simulink model "convertidor_inversor"  (R2022b)
settings: Solver=VariableStepAuto  StartTime=0.0  StopTime=1  RelTol=1e-3
InitFcn:
  | Ts = 100e-6;
StartFcn:
  | Ts = 100e-6;
undefined symbols (not defined in the file): Ion, Lithium
libraries: spsIGBTDiodeLib x8, slpidlib x7, spsCurrentMeasurementLib x5, spsVoltageMeasurementLib x5, spsThreePhaseSeriesRLCBranchLib x5, spsSeriesRLCBranchLib x4, spsAlphaBetaZerotodq0Lib x3, simulink x3, spsabctoAlphaBetaZeroLib x3, spsDCVoltageSourceLib x2, spsThreePhaseVIMeasurementLib x2, spsBatteryLib x1
(part 1 of 2)
settings Model: Creator=JGC  LastModifiedBy=ATV
settings SolverCC: AlgebraicLoopSolver=TrustRegion
settings DataIOCC: ReturnWorkspaceOutputs=off
settings DebuggingCC: UnconnectedInputMsg=warning  UnconnectedOutputMsg=warning  UnconnectedLineMsg=warning  SFMachineParentedDataDiag=warning
settings ModelReferenceCC: EnableRefExpFcnMdlSchedulingChecks=on
settings RTWCC: DLArmComputeVersion=19.05

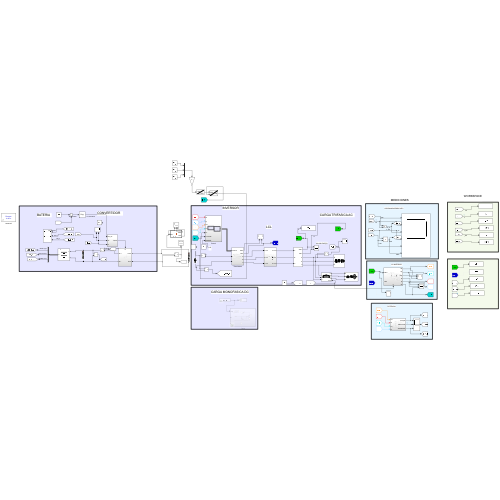
[thumbnail: Simulink's stored preview of the top-level diagram]
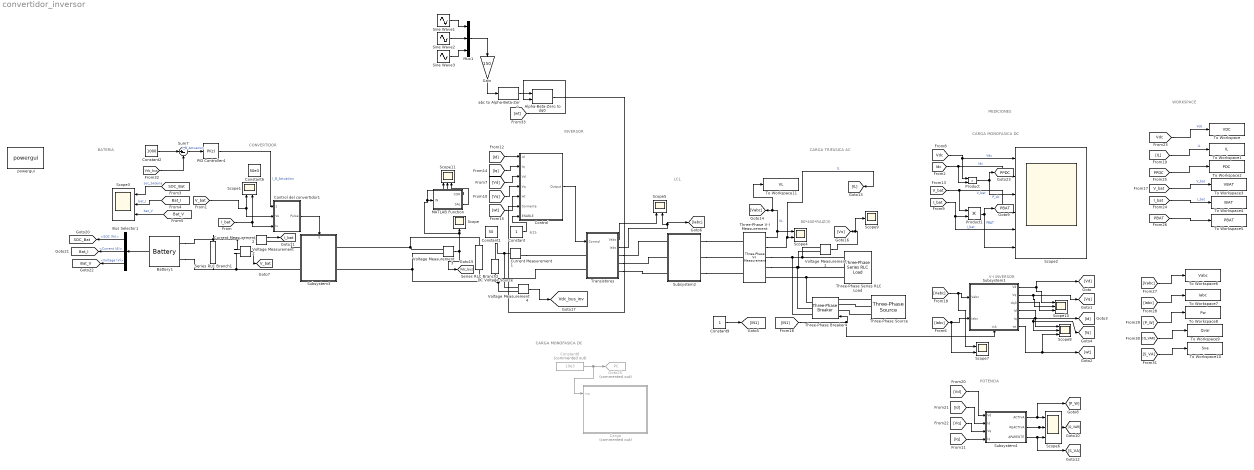
== system convertidor_inversor ==
  note: CARGA MONOFASICA DC
  note: CARGA TRIFASICA AC
  note: LCL
  note: INVERSOR
  note: MEDICIONES
  note: CARGA MONOFASICA DC
  note: BATERIA
  note: 80*400*RAIZ(3)
  note: 615
  note: POTENCIA
  note: V-I INVERSOR
  note: CONVERTIDOR
  note: WORKSPACE
  Alpha-Beta-Zero to dq0 : spsAlphaBetaZerotodq0Lib/Alpha-Beta-Zero to dq0  Alignment=90 degrees behind phase A axis
  Battery1 : spsBatteryLib/Battery  BatType=Lithium-Ion  ShowTempParam=off  ThermalPreset=no  ShowAgeParam=off  NomV=Battery.Nominal_voltage  NomQ=Battery.Rated_capacity  SOC=Battery.inicial_state_of_charge  Batt_Tr=Battery.response_time  PresetModel=on  MaxQ=200  MinV=384  FullV=595.9614  Dis_rate=86.9565  R=0.0256  Normal_OP=180.8696  expZone="[553.1576      9.826087]"  current=[6.5 7 100]  Units=Time  Tci=20  NomT=20  T2=-30  MaxQ2=4.8  FullV2=7.1  Normal_OP2=5.655  expZone2="[6.58           1]"  Rca=0.6  ti=2000  Dp=0  Neq0=0  Tsim=1e6  Ta1=25  Qeol=5.4*0.9  Reol=0.013333*1.2  Char_age=[2.3478, 3]  Dis_age=[2.3478, 10]  N1=1500  N2=10500  N3=1000  N4=1400  Ta2=45  N5=950
      settings: LibrarySourceBlock=electricdrivelib/Extra Sources/Battery
  Bus Selector1 : BusSelector  OutputSignals=SOC (%),Current (A),Voltage (V)
  Carga : Subsystem  Commented=on
  Constant : Constant
  Constant1 : Constant  Value=50
  Constant2 : Constant  Value=1000
  Constant6 : Constant  Value=50e3
  Constant8 : Constant  Commented=on  Value=10e3
  Constant9 : Constant
  "Control " : Subsystem
  Control del convertidor1 : Subsystem
  Current Measurement1 : spsCurrentMeasurementLib/Current Measurement  PhasorSimulation=off  OutputType=Complex  PSBequivalent=0
  Current Measurement2 : spsCurrentMeasurementLib/Current Measurement  PhasorSimulation=off  OutputType=Complex  PSBequivalent=0
  DC Voltage Source : spsDCVoltageSourceLib/DC Voltage Source  Amplitude=615  Measurements=None
  Gain : Gain  Gain=150
  Goto25 : Goto  Commented=on  GotoTag=PC  TagVisibility=global
  MATLAB Function : MATLAB Function  TreatAsAtomicUnit=on
  Mux1 : Mux  Inputs=3
  PID Controller4 : slpidlib/PID Controller  Controller=PI  Form=Parallel  TimeDomain=Discrete-time  UseExternalTs=off  SampleTime=Ts  IntegratorMethod=Forward Euler  FilterMethod=Forward Euler  ControllerParametersSource=internal  P=60  I=600  UseKiTs=off  D=0  N=100  UseFilter=on  TunerSelectOption=Transfer Function Based (PID Tuner App)  InitialConditionSource=internal  InitialConditionForIntegrator=0  InitialConditionForFilter=0  DifferentiatorICPrevScaledInput=0  ExternalReset=none  TrackingMode=off  Kt=1  LimitOutput=off  SatLimitsSource=internal  UpperSaturationLimit=0.95  LowerSaturationLimit=0  LinearizeAsGain=on  AntiWindupMode=clamping  Kb=1  LimitIntegrator=off  UpperIntegratorSaturationLimit=inf  LowerIntegratorSaturationLimit=-inf  POutMin=[]  POutMax=[]  IOutMin=[]  IOutMax=[]  DOutMin=[]  DOutMax=[]  NOutMin=[]  NOutMax=[]  SumOutMin=[]  SumOutMax=[]  SaturationOutMin=[]  SaturationOutMax=[]  PParamMin=[]  PParamMax=[]  IParamMin=[]  IParamMax=[]  DParamMin=[]  DParamMax=[]  NParamMin=[]  NParamMax=[]  KbParamMin=[]  KbParamMax=[]  KtParamMin=[]  KtParamMax=[]  KbOutMin=[]  KbOutMax=[]  KtOutMin=[]  KtOutMax=[]  IntegratorOutMin=[]  IntegratorOutMax=[]  FilterOutMin=[]  FilterOutMax=[]  SumI1OutMin=[]  SumI1OutMax=[]  SumI2OutMin=[]  SumI2OutMax=[]  SumI3OutMin=[]  SumI3OutMax=[]  SumI4OutMin=[]  SumI4OutMax=[]  SumDOutMin=[]  SumDOutMax=[]  DifferentiatorOutMin=[]  DifferentiatorOutMax=[]  FilterDiffOutCoefMin=[]  FilterDiffOutCoefMax=[]  ReciprocalOutMin=[]  ReciprocalOutMax=[]  SumDenOutMin=[]  SumDenOutMax=[]  SumNumOutMin=[]  SumNumOutMax=[]  DivideOutMin=[]  DivideOutMax=[]  UdiffTsProdOutMin=[]  UdiffTsProdOutMax=[]  NTsProdOutMin=[]  NTsProdOutMax=[]  UintegralTsProdOutMin=[]  UintegralTsProdOutMax=[]  UngainTsProdOutMin=[]  UngainTsProdOutMax=[]  ClampingZeroOutDataTypeStr=Inherit: Inherit via back propagation  ClampingZeroOutMin=[]  ClampingZeroOutMax=[]  FilterDenConstantOutDataTypeStr=Inherit: Inherit via back propagation  FilterDenConstantOutMin=[]  FilterDenConstantOutMax=[]  PCopyOutDataTypeStr=Inherit: Inherit via back propagation  PCopyOutMin=[]  PCopyOutMax=[]  NCopyOutDataTypeStr=Inherit: Inherit via back propagation  NCopyOutMin=[]  NCopyOutMax=[]  IntegratorContinuousStateAttributes=''  IntegratorStateMustResolveToSignalObject=off  IntegratorRTWStateStorageClass=Auto  FilterContinuousStateAttributes=''  FilterStateMustResolveToSignalObject=off  FilterRTWStateStorageClass=Auto  ParallelPVariant=InternalParameters  IdealPVariant=Disabled  IVariant=InternalParameters  DVariant=Disabled  IntegratorVariant=Discrete  SatVariant=Disabled  AWVariant=Passthrough  PCopyVariant=Disabled  TRVariant=Disabled  FdbkBlocksVariant=Forward  IdealPFdbkVariant=Disabled  SatFdbkVariant=Disabled  DerivativeFilterVariant=Disabled  NVariant=Disabled  NCopyVariant=Disabled_SignalSpec  FilterICVariant=Disabled  IntegratorICVariant=InternalICs  ExternalResetVariant=Disabled  TRSumVariant=Passthrough  SumFdbkVariant=Disabled  SumVariant=Sum_PI  TsampFilterVariant=InternalTs  TsampNgainVariant=Passthrough  TsampIntegralVariant=Passthrough  ExternalSaturationOutDataTypeStr=Inherit: Same as second input
  Product : Product
  Product1 : Product
  Scope : Scope
  Scope{1,4..5,7} (4 alike) : Scope  NumInputPorts=2
  Scope{3,6,8,10..11} (5 alike) : Scope  NumInputPorts=3
  Scope2 : Scope  NumInputPorts=6
  Scope9 : Scope
  Series RLC Branch1 : spsSeriesRLCBranchLib/Series RLC Branch  LConnTagsString=__new0  RConnTagsString=__new0  BranchType=RC  Resistance=0.3  Inductance=1e-3  SetiL0=off  InitialCurrent=0  Capacitance=1e-6  Setx0=on  InitialVoltage=512  Measurements=None
  Series RLC Branch2 : spsSeriesRLCBranchLib/Series RLC Branch  LConnTagsString=__new0  RConnTagsString=__new0  BranchType=C  Resistance=0.2  Inductance=1e-3  SetiL0=off  InitialCurrent=0  Capacitance=1000e-6  Setx0=on  InitialVoltage=400  Measurements=None
  Sine Wave1 : Sin  Frequency=2*pi*50  SampleTime=Ts
  Sine Wave2 : Sin  Frequency=2*pi*50  Phase=-120*2*pi/360  SampleTime=Ts
  Sine Wave3 : Sin  Frequency=2*pi*50  Phase=120*2*pi/360  SampleTime=Ts
  Subsystem1 : Subsystem
      settings: PortSchema="{\"entries\":[{\"content\":{\"sides\":[{\"content\":{\"connectorIds\":[\"In1\",\"In2\"]},\"type\":\"ConnectorPlacement.EquallySpacedRectSide\",\"uuid\":\"6be78711-4f19-4216-8280-237e362f2f67\"},{\"content\":{\"connectorIds\":[\"Out1\",\"Out2\",\"Out3\",\"Out4\",\"Out5\",\"Out6\"],\"side\":\"RIGHT\"},\"type\":\"ConnectorPlacement.EquallySpacedRectSide\",\"uuid\":\"8d48e04c-a554-48a1-8f05-ac010a5803c1\"},{\"content\":{\"connectorIds\":[],\"side\":\"TOP\"},\"type\":\"ConnectorPlacement.EquallySpacedRectSide\",\"uuid\":\"0ffbfd7d-1930-4ad5-9982-8469f3a97706\"},{\"content\":{\"connectorIds\":[\"In3\"],\"side\":\"BOTTOM\"},\"type\":\"ConnectorPlacement.EquallySpacedRectSide\",\"uuid\":\"6c965d76-c4d6-4dc7-a84d-e506f80fe6fe\"}]},\"type\":\"ConnectorPlacement.EquallySpacedConnector\",\"uuid\":\"0d915b79-5115-4aee-9d8b-435daa5fa966\"}],\"packageUris\":[\"http://schema.mathworks.com/mf0/Connector/R2020b\"],\"version\":\"1.0\"}"
  Subsystem2 : Subsystem
  Subsystem3 : Subsystem
      settings: PortSchema="{\"entries\":[{\"content\":{\"sides\":[{\"content\":{\"connectorIds\":[\"LConn1\",\"LConn2\"]},\"type\":\"ConnectorPlacement.EquallySpacedRectSide\",\"uuid\":\"7a980847-0fd3-4a52-ae22-59cd2a1ed559\"},{\"content\":{\"connectorIds\":[\"RConn1\",\"RConn2\"],\"side\":\"RIGHT\"},\"type\":\"ConnectorPlacement.EquallySpacedRectSide\",\"uuid\":\"85effeeb-73a6-4b0a-b51b-5eb0082317ff\"},{\"content\":{\"connectorIds\":[\"In1\"],\"side\":\"TOP\"},\"type\":\"ConnectorPlacement.EquallySpacedRectSide\",\"uuid\":\"eb55fae0-79ad-414f-ab96-49c332138803\"},{\"content\":{\"connectorIds\":[],\"side\":\"BOTTOM\"},\"type\":\"ConnectorPlacement.EquallySpacedRectSide\",\"uuid\":\"1fd972ff-419a-4657-8ea4-57d89be2b868\"}]},\"type\":\"ConnectorPlacement.EquallySpacedConnector\",\"uuid\":\"1807473d-fd42-44e0-a7e4-668a7bf21429\"}],\"packageUris\":[\"http://schema.mathworks.com/mf0/Connector/R2020b\"],\"version\":\"1.0\"}"
  Subsystem4 : Subsystem
  Sum7 : Sum  Inputs=|+-
  Three-Phase Series RLC Load : spsThreePhaseSeriesRLCLoadLib/Three-Phase Series RLC Load  LConnTagsString=A|B|C  Configuration=Y (grounded)  NominalVoltage=400  Vabc=[1e3 1e3 1e3]  Vabcp=[1e3 1e3 1e3]  NominalFrequency=50  UnbalancedPower=off  ActivePower=50e3  InductivePower=100  CapacitivePower=100  Pabc=[10e3 9e3 11e3]  QLabc=[100 90 110]  QCabc=[100 90 110]  Pabcp=[10e3 9e3 11e3]  QLabcp=[100 90 110]  QCabcp=[100 90 110]  Measurements=None  LoadType=constant Z
  Three-Phase V-I Measurement : spsThreePhaseVIMeasurementLib/Three-Phase V-I Measurement  VoltageMeasurement=phase-to-phase  SetLabelV=off  LabelV=Vabc  Vpu=off  VpuLL=off  CurrentMeasurement=yes  SetLabelI=off  LabelI=Iabc  Ipu=off  Pbase=100e6  Vbase=500e3  OutputType=Complex  PhasorSimulation=off  PSBequivalent=0
  Three-Phase Breaker4 : spsThreePhaseBreakerLib/Three-Phase Breaker  InitialState=closed  SwitchA=on  SwitchB=on  SwitchC=on  SwitchTimes="[1/60  5/60]"  External=on  BreakerResistance=0.01  SnubberResistance=1e6  SnubberCapacitance=inf  Measurements=None
  Three-Phase Source : spsThreePhaseSourceLib/Three-Phase Source  InternalConnection=Y  VoltagePhases=off  Voltage=400  PhaseAngle=0  Voltage_phases=[25e3 25e3 25e3]/sqrt(3)  PhaseAngles_phases=[0 -120 +120]  Frequency=50  NonIdealSource=on  SpecifyImpedance=off  Resistance=0.0001e-3  Inductance=0.0001e-9  ShortCircuitLevel=100e6  BaseVoltage=400  XRratio=7  BusType=swing  Pref=10e3  Qref=0  Prefabc=[10e3, 10e3, 10e3]  Qrefabc=[0, 0, 0]  Qmin=-inf  Qmax=inf
  To Workspace : ToWorkspace  VariableName=VDC  SaveFormat=Timeseries  SampleTime=-1
  To Workspace1 : ToWorkspace  VariableName=IL  SaveFormat=Timeseries  SampleTime=-1
  To Workspace10 : ToWorkspace  VariableName=Sva  SaveFormat=Timeseries  SampleTime=-1
  To Workspace11 : ToWorkspace  VariableName=VL  SaveFormat=Timeseries  SampleTime=-1
  To Workspace2 : ToWorkspace  VariableName=PDC  SaveFormat=Timeseries  SampleTime=-1
  To Workspace3 : ToWorkspace  VariableName=VBAT  SaveFormat=Timeseries  SampleTime=-1
  To Workspace4 : ToWorkspace  VariableName=IBAT  SaveFormat=Timeseries  SampleTime=-1
  To Workspace5 : ToWorkspace  VariableName=PBAT  SaveFormat=Timeseries  SampleTime=-1
  To Workspace6 : ToWorkspace  VariableName=Vabc  SaveFormat=Timeseries  SampleTime=-1
  To Workspace7 : ToWorkspace  VariableName=Iabc  SaveFormat=Timeseries  SampleTime=-1
  To Workspace8 : ToWorkspace  VariableName=Pw  SaveFormat=Timeseries  SampleTime=-1
  To Workspace9 : ToWorkspace  VariableName=Qvar  SaveFormat=Timeseries  SampleTime=-1
  Transistores : Subsystem
  Voltage Measurement{1..4} (4 alike) : spsVoltageMeasurementLib/Voltage Measurement  PhasorSimulation=off  OutputType=Complex  PSBequivalent=0
  abc to Alpha-Beta-Zero : spsabctoAlphaBetaZeroLib/abc to Alpha-Beta-Zero
  powergui : sps_lib/powergui  Priority=1  SimulationMode=Discrete  SampleTime=1e-5  frequency=60  Iterations=50  frequencyindice=0  Pbase=100e6  ErrMax=1e-4  UnitsV=kV  UnitsW=MW  buscounter=0  FunctionMessages=off  echomessages=off  EnableUseOfTLC=off  CurrentSourceSwitches=off  DisableSnubberDevices=off  DisableRonSwitches=off  DisableVfSwitches=off  DisplayEquations=off  AutomaticDiscreteSolvers=off  SolverType=Tustin/Backward Euler (TBE)  Interpol=off  ExternalGateDelay=off  methode=off  Ts=100  x0status=blocks  SPID=on  SwTol=0  HookPort=off  NonlinearTolerance=1e-4  nMaxIteration=100  ContinueOnMaxIteration=off  RestoreLinks=warning  ResistiveCurrentMeasurement=off  Frange=[0:2:500]  Ylog=off  Xlog=on  ShowGrid=off  save=off  variable=ZData  structure=logsout  ZoomFFT=off  StartTime=0.02  cycles=8  DisplayStyle=1  fundamental=50  FreqAxis=off  MaxFrequency=1000  frequencyindicesteady=1  RmsSteady=1  display=off
  tag scope: Bat_I=global, Bat_V=global, I_bat=global, PBAT=global, PPDC=global, SOC_Bat=global, V_bat=global, Vdc_bus=global, Vdc_bus_inv=global
  wires:
  Voltage Measurement2/1 -> [V_bat]
  Bus Selector1/3 -> [Bat_V]  "<Voltage (V)>"
  [SOC_Bat] -> Scope3/1  "soc_bateria"
  Control del convertidor1/1(Pulse) -> Subsystem3/1(S)
  Current Measurement2/1 -> [I_bat]
  [Bat_I] -> Scope3/2  "bat_I"
  [I_bat] -> Control del convertidor1/3(Is), Scope1/2
  [Bat_V] -> Scope3/3  "bat_V"
  Bus Selector1/1 -> [SOC_Bat]  "<SOC (%)>"
  Battery1/1 -> Bus Selector1/1
  [V_bat] -> Control del convertidor1/2(Vs), Scope1/1
  Bus Selector1/2 -> [Bat_I]  "<Current (A)>"
  Constant8/1 -> Goto25/1, Carga/1(vvp)
  Product/1 -> [PPDC], Scope2/3  "P_dc"
  Product1/1 -> [PBAT], Scope2/6  "PBAT"
  [V_bat] -> Product1/1, Scope2/4  "V_bat"
  [I_bat] -> Scope2/5, Product1/2  "I_bat"
  [Vdc] -> Scope2/1, Product/1  "Vdc"
  [Idc] -> Scope2/2, Product/2  "Idc"
  [wt] -> "Control "/5(wt)
  [Id] -> Subsystem4/2(Id)
  Subsystem1/5(Iq) -> Scope8/2, [Iq]
  [Vd] -> Subsystem4/1(Vd)
  "Control "/1(Output) -> Transistores/1(Control)
  [Iq] -> Subsystem4/4(Iq)
  [Iabc] -> Scope7/2, Subsystem1/2(Iabc)
  Subsystem1/6(wt) -> Scope8/3, [wt]
  Three-Phase V-I Measurement/1 -> To Workspace11/1, [Vabc], Scope4/1  "VL"
  Subsystem1/1(Vd) -> Scope10/1, [Vd]
  Subsystem1/2(Vq) -> Scope10/2, [Vq]
  Subsystem1/4(Id) -> [Id], Scope8/1
  [Vq] -> Subsystem4/3(Vq)
  Subsystem1/3(dq0) -> Scope10/3
  Transistores/2(Iabc) -> Scope5/2, [Iabc]
  Transistores/1(Vabc) -> Scope5/1
  Three-Phase V-I Measurement/2 -> [IL], Scope4/2  "IL"
  [Vabc] -> Scope7/1, Subsystem1/1(Vabc)
  [Vq] -> "Control "/4(Vq)
  [Iq] -> "Control "/2(Iq)
  [Vd] -> "Control "/3(Vd)
  [Id] -> "Control "/1(Id)
  Subsystem4/1(ACTIVA) -> [P_W], Scope6/1
  Subsystem4/2(REACTIVA) -> [Q_VAR], Scope6/2
  Subsystem4/3(APARENTE) -> [S_VA], Scope6/3
  Voltage Measurement3/1 -> Scope11/1, MATLAB Function/1(IN), Scope/1, [Vdc_bus]
  [IN1] -> Subsystem1/3(In3), Three-Phase Breaker4/1
  Constant9/1 -> [IN1]
  [Vdc] -> To Workspace/1  "Vdc"
  [IL] -> To Workspace1/1  "IL"
  [PPDC] -> To Workspace2/1
  [V_bat] -> To Workspace3/1  "V_bat"
  [I_bat] -> To Workspace4/1  "I_bat"
  [PBAT] -> To Workspace5/1
  [Vabc] -> To Workspace6/1
  [Iabc] -> To Workspace7/1
  [P_W] -> To Workspace8/1
  [Q_VAR] -> To Workspace9/1
  [S_VA] -> To Workspace10/1
  Voltage Measurement1/1 -> Scope9/1, [Vo]
  MATLAB Function/1(COR) -> Scope11/2
  MATLAB Function/2(SAL) -> Scope11/3
  Sum7/1 -> PID Controller4/1  "I_B_Actuation"
  Constant2/1 -> Sum7/1
  PID Controller4/1 -> Control del convertidor1/1(Pot_ref)  "I_B_Actuation"
  [Vdc_bus] -> Sum7/2
  Constant/1 -> "Control "/7(ENABLE)
  Voltage Measurement4/1 -> [Vdc_bus_inv]
  abc to Alpha-Beta-Zero/1 -> Alpha-Beta-Zero to dq0/1
  [wt] -> Alpha-Beta-Zero to dq0/2
  Alpha-Beta-Zero to dq0/1 -> "Control "/6(Corriente)
  Sine Wave3/1 -> Mux1/3
  Sine Wave1/1 -> Mux1/1
  Sine Wave2/1 -> Mux1/2
  Mux1/1 -> Gain/1
  Gain/1 -> abc to Alpha-Beta-Zero/1
  connections:
  Voltage Measurement2/LConn2 -- Series RLC Branch1/RConn1 -- Battery1/LConn2 -- Subsystem3/LConn2
  Battery1/LConn1 -- Current Measurement2/LConn1 -- Voltage Measurement2/LConn1 -- Series RLC Branch1/LConn1
  Subsystem3/LConn1 -- Current Measurement2/RConn1
  Three-Phase V-I Measurement/RConn2 -- Three-Phase Breaker4/RConn2 -- Three-Phase Series RLC Load/LConn2 -- Voltage Measurement1/LConn2
  Three-Phase V-I Measurement/RConn1 -- Three-Phase Breaker4/RConn1 -- Voltage Measurement1/LConn1 -- Three-Phase Series RLC Load/LConn1
  Three-Phase Series RLC Load/LConn3 -- Three-Phase Breaker4/RConn3 -- Three-Phase V-I Measurement/RConn3
  Series RLC Branch2/LConn1 -- Subsystem3/RConn1 -- Voltage Measurement3/LConn1
  Subsystem2/LConn2 -- Three-Phase V-I Measurement/LConn2
  Subsystem2/LConn1 -- Three-Phase V-I Measurement/LConn1
  Transistores/RConn1 -- Subsystem2/RConn1
  Transistores/RConn3 -- Subsystem2/RConn3
  Transistores/LConn2 -- Voltage Measurement4/LConn2 -- DC Voltage Source/LConn1
  Subsystem2/LConn3 -- Three-Phase V-I Measurement/LConn3
  Transistores/RConn2 -- Subsystem2/RConn2
  Three-Phase Source/RConn1 -- Three-Phase Breaker4/LConn1
  Three-Phase Source/RConn2 -- Three-Phase Breaker4/LConn2
  Three-Phase Source/RConn3 -- Three-Phase Breaker4/LConn3
  Current Measurement1/RConn1 -- Transistores/LConn1
  Current Measurement1/LConn1 -- Voltage Measurement4/LConn1 -- DC Voltage Source/RConn1
  Series RLC Branch2/RConn1 -- Voltage Measurement3/LConn2 -- Subsystem3/RConn2

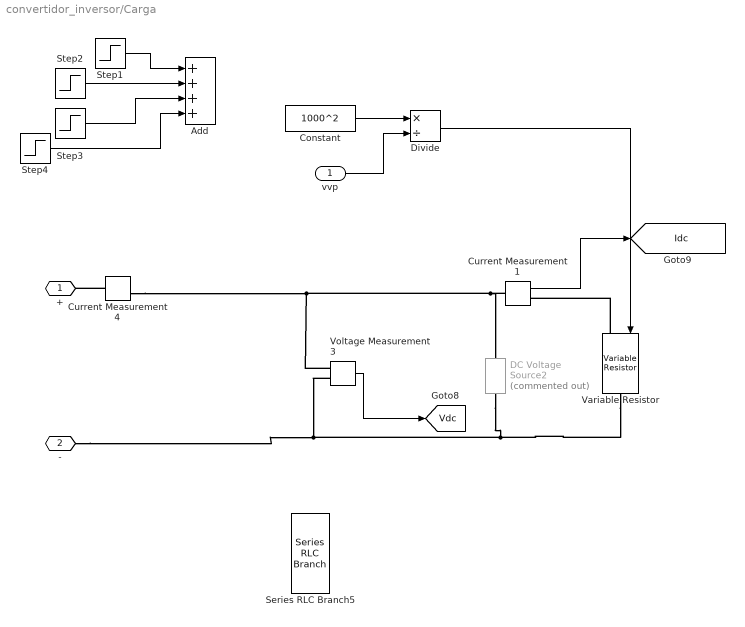
== system convertidor_inversor/Carga ==
  vvp : Inport
  Add : Sum  Inputs=++++
  Constant : Constant  Value=1000^2
  Current Measurement1 : spsCurrentMeasurementLib/Current Measurement  PhasorSimulation=off  OutputType=Complex  PSBequivalent=0
  Current Measurement4 : spsCurrentMeasurementLib/Current Measurement  PhasorSimulation=off  OutputType=Complex  PSBequivalent=0
  DC Voltage Source2 : spsDCVoltageSourceLib/DC Voltage Source  Commented=on  Amplitude=800  Measurements=None
  Divide : Product  Inputs=*/
  Series RLC Branch5 : spsSeriesRLCBranchLib/Series RLC Branch  LConnTagsString=__new0  RConnTagsString=__new0  BranchType=C  Resistance=0.2  Inductance=1e-3  SetiL0=off  InitialCurrent=0  Capacitance=300e-6  Setx0=on  InitialVoltage=512  Measurements=None
  Step1 : Step  After=5000  SampleTime=0
  Step2 : Step  Time=2  After=-7500  SampleTime=0
  Step3 : Step  Time=3  After=10000  SampleTime=0
  Step4 : Step  Time=4  After=-7500  SampleTime=0
  Variable Resistor : spsVariableResistorLib/Variable Resistor  Rabsmin=1e-3
      settings: LibrarySourceBlock=sps_lib/Passives/Variable Resistor
  Voltage Measurement3 : spsVoltageMeasurementLib/Voltage Measurement  PhasorSimulation=off  OutputType=Complex  PSBequivalent=0
  + : PMIOPort  Side=Left
  - : PMIOPort  Port=2  Side=Left
  tag scope: Idc=global, Vdc=global
  wires:
  Voltage Measurement3/1 -> [Vdc]
  Constant/1 -> Divide/1
  Divide/1 -> Variable Resistor/1
  Step1/1 -> Add/1
  Step2/1 -> Add/2
  Step3/1 -> Add/3
  Step4/1 -> Add/4
  Current Measurement1/1 -> [Idc]
  vvp/1 -> Divide/2
  connections:
  Voltage Measurement3/LConn2 -- -/RConn1 -- Variable Resistor/RConn1 -- DC Voltage Source2/LConn1
  Current Measurement4/LConn1 -- +/RConn1
  Variable Resistor/LConn1 -- Current Measurement1/RConn1
  Current Measurement4/RConn1 -- Voltage Measurement3/LConn1 -- DC Voltage Source2/RConn1 -- Current Measurement1/LConn1

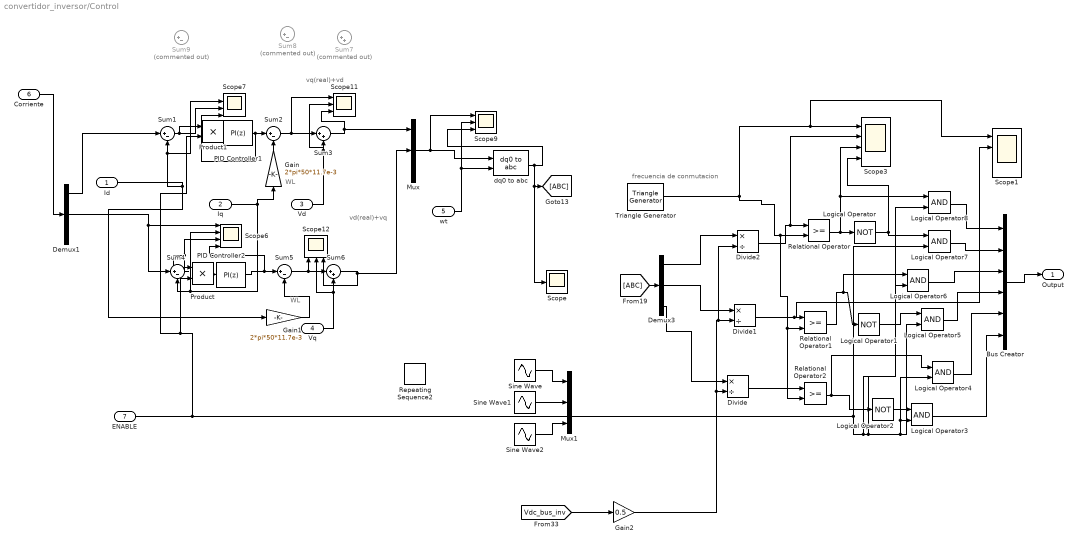
== system convertidor_inversor/Control  ==
  note: frecuencia de conmutacion
  note: WL
  note: WL
  note: vq(real)+vd
  note: vd(real)+vq
  Id : Inport
  Iq : Inport  Port=2
  Vd : Inport  Port=3
  Vq : Inport  Port=4
  wt : Inport  Port=5
  Corriente : Inport  Port=6
  ENABLE : Inport  Port=7
  Bus Creator : BusCreator  Inputs=6
  Demux1 : Demux  Outputs=3
  Demux3 : Demux  Outputs=3
  Divide : Product  Inputs=*/
  Divide1 : Product  Inputs=*/
  Divide2 : Product  Inputs=*/
  Gain : Gain  Gain=2*pi*50*11.7e-3
  Gain1 : Gain  Gain=2*pi*50*11.7e-3
  Gain2 : Gain  Gain=0.5
  Logical Operator : Logic  Operator=NOT  AllPortsSameDT=off  OutDataTypeStr=boolean
  Logical Operator1 : Logic  Operator=NOT  AllPortsSameDT=off  OutDataTypeStr=boolean
  Logical Operator2 : Logic  Operator=NOT  AllPortsSameDT=off  OutDataTypeStr=boolean
  Logical Operator{3..8} (6 alike) : Logic  AllPortsSameDT=off  OutDataTypeStr=boolean
  Mux : Mux  Inputs=3
  Mux1 : Mux  Inputs=3
  PID Controller1 : slpidlib/PID Controller  Controller=PI  Form=Parallel  TimeDomain=Discrete-time  UseExternalTs=off  SampleTime=Ts  IntegratorMethod=Forward Euler  FilterMethod=Forward Euler  ControllerParametersSource=internal  P=60  I=0  UseKiTs=off  D=0  N=100  UseFilter=on  TunerSelectOption=Transfer Function Based (PID Tuner App)  InitialConditionSource=internal  InitialConditionForIntegrator=0  InitialConditionForFilter=0  DifferentiatorICPrevScaledInput=0  ExternalReset=none  TrackingMode=off  Kt=1  LimitOutput=off  SatLimitsSource=internal  UpperSaturationLimit=inf  LowerSaturationLimit=-inf  LinearizeAsGain=on  AntiWindupMode=none  Kb=1  LimitIntegrator=off  UpperIntegratorSaturationLimit=inf  LowerIntegratorSaturationLimit=-inf  POutMin=[]  POutMax=[]  IOutMin=[]  IOutMax=[]  DOutMin=[]  DOutMax=[]  NOutMin=[]  NOutMax=[]  SumOutMin=[]  SumOutMax=[]  SaturationOutMin=[]  SaturationOutMax=[]  PParamMin=[]  PParamMax=[]  IParamMin=[]  IParamMax=[]  DParamMin=[]  DParamMax=[]  NParamMin=[]  NParamMax=[]  KbParamMin=[]  KbParamMax=[]  KtParamMin=[]  KtParamMax=[]  KbOutMin=[]  KbOutMax=[]  KtOutMin=[]  KtOutMax=[]  IntegratorOutMin=[]  IntegratorOutMax=[]  FilterOutMin=[]  FilterOutMax=[]  SumI1OutMin=[]  SumI1OutMax=[]  SumI2OutMin=[]  SumI2OutMax=[]  SumI3OutMin=[]  SumI3OutMax=[]  SumI4OutMin=[]  SumI4OutMax=[]  SumDOutMin=[]  SumDOutMax=[]  DifferentiatorOutMin=[]  DifferentiatorOutMax=[]  FilterDiffOutCoefMin=[]  FilterDiffOutCoefMax=[]  ReciprocalOutMin=[]  ReciprocalOutMax=[]  SumDenOutMin=[]  SumDenOutMax=[]  SumNumOutMin=[]  SumNumOutMax=[]  DivideOutMin=[]  DivideOutMax=[]  UdiffTsProdOutMin=[]  UdiffTsProdOutMax=[]  NTsProdOutMin=[]  NTsProdOutMax=[]  UintegralTsProdOutMin=[]  UintegralTsProdOutMax=[]  UngainTsProdOutMin=[]  UngainTsProdOutMax=[]  ClampingZeroOutDataTypeStr=Inherit: Inherit via back propagation  ClampingZeroOutMin=[]  ClampingZeroOutMax=[]  FilterDenConstantOutDataTypeStr=Inherit: Inherit via back propagation  FilterDenConstantOutMin=[]  FilterDenConstantOutMax=[]  PCopyOutDataTypeStr=Inherit: Inherit via back propagation  PCopyOutMin=[]  PCopyOutMax=[]  NCopyOutDataTypeStr=Inherit: Inherit via back propagation  NCopyOutMin=[]  NCopyOutMax=[]  IntegratorContinuousStateAttributes=''  IntegratorStateMustResolveToSignalObject=off  IntegratorRTWStateStorageClass=Auto  FilterContinuousStateAttributes=''  FilterStateMustResolveToSignalObject=off  FilterRTWStateStorageClass=Auto  ParallelPVariant=InternalParameters  IdealPVariant=Disabled  IVariant=InternalParameters  DVariant=Disabled  IntegratorVariant=Discrete  SatVariant=Disabled  AWVariant=Passthrough  PCopyVariant=Disabled  TRVariant=Disabled  FdbkBlocksVariant=Forward  IdealPFdbkVariant=Disabled  SatFdbkVariant=Disabled  DerivativeFilterVariant=Disabled  NVariant=Disabled  NCopyVariant=Disabled_SignalSpec  FilterICVariant=Disabled  IntegratorICVariant=InternalICs  ExternalResetVariant=Disabled  TRSumVariant=Passthrough  SumFdbkVariant=Disabled  SumVariant=Sum_PI  TsampFilterVariant=InternalTs  TsampNgainVariant=Passthrough  TsampIntegralVariant=Passthrough  ExternalSaturationOutDataTypeStr=Inherit: Same as second input
  PID Controller2 : slpidlib/PID Controller  Controller=PI  Form=Parallel  TimeDomain=Discrete-time  UseExternalTs=off  SampleTime=Ts  IntegratorMethod=Forward Euler  FilterMethod=Forward Euler  ControllerParametersSource=internal  P=50  I=0  UseKiTs=off  D=0  N=100  UseFilter=on  TunerSelectOption=Transfer Function Based (PID Tuner App)  InitialConditionSource=internal  InitialConditionForIntegrator=0  InitialConditionForFilter=0  DifferentiatorICPrevScaledInput=0  ExternalReset=none  TrackingMode=off  Kt=1  LimitOutput=off  SatLimitsSource=internal  UpperSaturationLimit=inf  LowerSaturationLimit=-inf  LinearizeAsGain=on  AntiWindupMode=none  Kb=1  LimitIntegrator=off  UpperIntegratorSaturationLimit=inf  LowerIntegratorSaturationLimit=-inf  POutMin=[]  POutMax=[]  IOutMin=[]  IOutMax=[]  DOutMin=[]  DOutMax=[]  NOutMin=[]  NOutMax=[]  SumOutMin=[]  SumOutMax=[]  SaturationOutMin=[]  SaturationOutMax=[]  PParamMin=[]  PParamMax=[]  IParamMin=[]  IParamMax=[]  DParamMin=[]  DParamMax=[]  NParamMin=[]  NParamMax=[]  KbParamMin=[]  KbParamMax=[]  KtParamMin=[]  KtParamMax=[]  KbOutMin=[]  KbOutMax=[]  KtOutMin=[]  KtOutMax=[]  IntegratorOutMin=[]  IntegratorOutMax=[]  FilterOutMin=[]  FilterOutMax=[]  SumI1OutMin=[]  SumI1OutMax=[]  SumI2OutMin=[]  SumI2OutMax=[]  SumI3OutMin=[]  SumI3OutMax=[]  SumI4OutMin=[]  SumI4OutMax=[]  SumDOutMin=[]  SumDOutMax=[]  DifferentiatorOutMin=[]  DifferentiatorOutMax=[]  FilterDiffOutCoefMin=[]  FilterDiffOutCoefMax=[]  ReciprocalOutMin=[]  ReciprocalOutMax=[]  SumDenOutMin=[]  SumDenOutMax=[]  SumNumOutMin=[]  SumNumOutMax=[]  DivideOutMin=[]  DivideOutMax=[]  UdiffTsProdOutMin=[]  UdiffTsProdOutMax=[]  NTsProdOutMin=[]  NTsProdOutMax=[]  UintegralTsProdOutMin=[]  UintegralTsProdOutMax=[]  UngainTsProdOutMin=[]  UngainTsProdOutMax=[]  ClampingZeroOutDataTypeStr=Inherit: Inherit via back propagation  ClampingZeroOutMin=[]  ClampingZeroOutMax=[]  FilterDenConstantOutDataTypeStr=Inherit: Inherit via back propagation  FilterDenConstantOutMin=[]  FilterDenConstantOutMax=[]  PCopyOutDataTypeStr=Inherit: Inherit via back propagation  PCopyOutMin=[]  PCopyOutMax=[]  NCopyOutDataTypeStr=Inherit: Inherit via back propagation  NCopyOutMin=[]  NCopyOutMax=[]  IntegratorContinuousStateAttributes=''  IntegratorStateMustResolveToSignalObject=off  IntegratorRTWStateStorageClass=Auto  FilterContinuousStateAttributes=''  FilterStateMustResolveToSignalObject=off  FilterRTWStateStorageClass=Auto  ParallelPVariant=InternalParameters  IdealPVariant=Disabled  IVariant=InternalParameters  DVariant=Disabled  IntegratorVariant=Discrete  SatVariant=Disabled  AWVariant=Passthrough  PCopyVariant=Disabled  TRVariant=Disabled  FdbkBlocksVariant=Forward  IdealPFdbkVariant=Disabled  SatFdbkVariant=Disabled  DerivativeFilterVariant=Disabled  NVariant=Disabled  NCopyVariant=Disabled_SignalSpec  FilterICVariant=Disabled  IntegratorICVariant=InternalICs  ExternalResetVariant=Disabled  TRSumVariant=Passthrough  SumFdbkVariant=Disabled  SumVariant=Sum_PI  TsampFilterVariant=InternalTs  TsampNgainVariant=Passthrough  TsampIntegralVariant=Passthrough  ExternalSaturationOutDataTypeStr=Inherit: Same as second input
  Product : Product
  Product1 : Product
  Relational Operator : RelationalOperator  OutDataTypeStr=boolean  RndMeth=Simplest  InputSameDT=off
  Relational Operator1 : RelationalOperator  OutDataTypeStr=boolean  RndMeth=Simplest  InputSameDT=off
  Relational Operator2 : RelationalOperator  OutDataTypeStr=boolean  RndMeth=Simplest  InputSameDT=off
  Repeating Sequence2 : simulink/Sources/Repeating Sequence  rep_seq_t=[0 Ts/2 Ts]  rep_seq_y=[0 1 0]
  Scope : Scope
  Scope{1,3,6..7} (4 alike) : Scope  NumInputPorts=4
  Scope11 : Scope  NumInputPorts=3
  Scope12 : Scope  NumInputPorts=3
  Scope9 : Scope  NumInputPorts=3
  Sine Wave : Sin  Amplitude=615/2  Frequency=2*pi*50  SampleTime=Ts
  Sine Wave1 : Sin  Amplitude=615/2  Frequency=2*pi*50  Phase=-120*2*pi/360  SampleTime=Ts
  Sine Wave2 : Sin  Amplitude=615/2  Frequency=2*pi*50  Phase=120*2*pi/360  SampleTime=Ts
  Sum{1..2,4..5} (4 alike) : Sum  Inputs=|+-
  Sum3 : Sum  Inputs=|++
  Sum6 : Sum  Inputs=|++
  Sum7 : Sum  Commented=on  Inputs=|++
  Sum8 : Sum  Commented=on  Inputs=|+-
  Sum9 : Sum  Commented=on  Inputs=|+-
  Triangle Generator : spsTriangleGeneratorLib/Triangle Generator  Freq=10e3  Phase=90  Ts=0
  dq0 to abc : spsdq0toabcLib/dq0 to abc  Alignment=90 degrees behind phase A axis
  Output : Outport
  wires:
  Gain1/1 -> Sum5/2
  Vq/1 -> Scope12/2, Sum6/2
  Demux3/2 -> Divide1/1
  Sum2/1 -> Scope11/1, Sum3/1
  Demux3/3 -> Divide/1
  PID Controller1/1 -> Scope7/4, Sum2/1
  Sum5/1 -> Scope12/1, Sum6/1
  Iq/1 -> Gain/1, Sum4/2, Scope6/2
  Gain/1 -> Sum2/2
  Id/1 -> Gain1/1, Scope7/2, Sum1/2
  Demux1/2 -> Sum4/1, Scope6/1
  PID Controller2/1 -> Scope6/4, Sum5/1
  Sum6/1 -> Mux/2, Scope12/3
  Sum3/1 -> Mux/1, Scope11/3
  Divide/1 -> Relational Operator2/1
  Divide1/1 -> Scope1/2, Relational Operator1/1
  Relational Operator2/1 -> Logical Operator4/1, Logical Operator2/1
  Relational Operator1/1 -> Logical Operator6/1, Logical Operator1/1
  dq0 to abc/1 -> Scope/1, [ABC], Scope9/3
  Triangle Generator/1 -> Relational Operator2/2, Relational Operator1/2, Relational Operator/2, Scope1/1, Scope3/1
  Sum1/1 -> Product1/1, Scope7/3
  wt/1 -> Scope9/2, dq0 to abc/2
  Sum4/1 -> Product/1, Scope6/3
  Vd/1 -> Scope11/2, Sum3/2
  Divide2/1 -> Scope3/2, Relational Operator/1
  Relational Operator/1 -> Logical Operator8/1, Scope3/3, Logical Operator/1
  Mux/1 -> Scope9/1, dq0 to abc/1
  Demux3/1 -> Divide2/1
  Logical Operator/1 -> Scope3/4, Logical Operator7/1
  Bus Creator/1 -> Output/1
  Logical Operator3/1 -> Bus Creator/6
  Logical Operator2/1 -> Logical Operator3/1
  Logical Operator4/1 -> Bus Creator/5
  Logical Operator1/1 -> Logical Operator5/1
  Logical Operator5/1 -> Bus Creator/4
  Logical Operator6/1 -> Bus Creator/3
  Logical Operator7/1 -> Bus Creator/2
  Logical Operator8/1 -> Bus Creator/1
  ENABLE/1 -> Product1/2, Product/2, Logical Operator6/2, Logical Operator8/2, Logical Operator5/2, Logical Operator4/2, Logical Operator3/2, Logical Operator7/2
  Product/1 -> PID Controller2/1
  [Vdc_bus_inv] -> Gain2/1
  Gain2/1 -> Divide2/2, Divide1/2, Divide/2
  Sine Wave1/1 -> Mux1/2
  Sine Wave/1 -> Mux1/1
  Sine Wave2/1 -> Mux1/3
  [ABC] -> Demux3/1
  Corriente/1 -> Demux1/1
  Demux1/1 -> Sum1/1

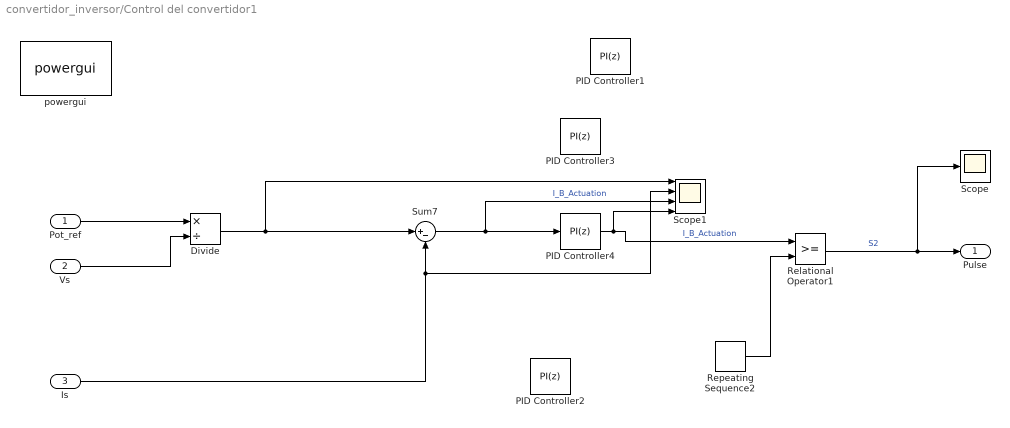
== system convertidor_inversor/Control del convertidor1 ==
  Pot_ref : Inport
  Vs : Inport  Port=2
  Is : Inport  Port=3
  Divide : Product  Inputs=*/
  PID Controller1 : slpidlib/PID Controller  Controller=PI  Form=Parallel  TimeDomain=Discrete-time  UseExternalTs=off  SampleTime=Ts  IntegratorMethod=Forward Euler  FilterMethod=Forward Euler  ControllerParametersSource=internal  P=0.01  I=0.02  UseKiTs=off  D=0  N=100  UseFilter=on  TunerSelectOption=Transfer Function Based (PID Tuner App)  InitialConditionSource=internal  InitialConditionForIntegrator=0  InitialConditionForFilter=0  DifferentiatorICPrevScaledInput=0  ExternalReset=none  TrackingMode=off  Kt=1  LimitOutput=on  SatLimitsSource=internal  UpperSaturationLimit=0.95  LowerSaturationLimit=0  LinearizeAsGain=on  AntiWindupMode=clamping  Kb=1  LimitIntegrator=off  UpperIntegratorSaturationLimit=inf  LowerIntegratorSaturationLimit=-inf  POutMin=[]  POutMax=[]  IOutMin=[]  IOutMax=[]  DOutMin=[]  DOutMax=[]  NOutMin=[]  NOutMax=[]  SumOutMin=[]  SumOutMax=[]  SaturationOutMin=[]  SaturationOutMax=[]  PParamMin=[]  PParamMax=[]  IParamMin=[]  IParamMax=[]  DParamMin=[]  DParamMax=[]  NParamMin=[]  NParamMax=[]  KbParamMin=[]  KbParamMax=[]  KtParamMin=[]  KtParamMax=[]  KbOutMin=[]  KbOutMax=[]  KtOutMin=[]  KtOutMax=[]  IntegratorOutMin=[]  IntegratorOutMax=[]  FilterOutMin=[]  FilterOutMax=[]  SumI1OutMin=[]  SumI1OutMax=[]  SumI2OutMin=[]  SumI2OutMax=[]  SumI3OutMin=[]  SumI3OutMax=[]  SumI4OutMin=[]  SumI4OutMax=[]  SumDOutMin=[]  SumDOutMax=[]  DifferentiatorOutMin=[]  DifferentiatorOutMax=[]  FilterDiffOutCoefMin=[]  FilterDiffOutCoefMax=[]  ReciprocalOutMin=[]  ReciprocalOutMax=[]  SumDenOutMin=[]  SumDenOutMax=[]  SumNumOutMin=[]  SumNumOutMax=[]  DivideOutMin=[]  DivideOutMax=[]  UdiffTsProdOutMin=[]  UdiffTsProdOutMax=[]  NTsProdOutMin=[]  NTsProdOutMax=[]  UintegralTsProdOutMin=[]  UintegralTsProdOutMax=[]  UngainTsProdOutMin=[]  UngainTsProdOutMax=[]  ClampingZeroOutDataTypeStr=Inherit: Inherit via back propagation  ClampingZeroOutMin=[]  ClampingZeroOutMax=[]  FilterDenConstantOutDataTypeStr=Inherit: Inherit via back propagation  FilterDenConstantOutMin=[]  FilterDenConstantOutMax=[]  PCopyOutDataTypeStr=Inherit: Inherit via back propagation  PCopyOutMin=[]  PCopyOutMax=[]  NCopyOutDataTypeStr=Inherit: Inherit via back propagation  NCopyOutMin=[]  NCopyOutMax=[]  IntegratorContinuousStateAttributes=''  IntegratorStateMustResolveToSignalObject=off  IntegratorRTWStateStorageClass=Auto  FilterContinuousStateAttributes=''  FilterStateMustResolveToSignalObject=off  FilterRTWStateStorageClass=Auto  ParallelPVariant=InternalParameters  IdealPVariant=Disabled  IVariant=InternalParameters  DVariant=Disabled  IntegratorVariant=Discrete  SatVariant=Enabled  AWVariant=DiscClampingParallel  PCopyVariant=Disabled  TRVariant=Disabled  FdbkBlocksVariant=Forward  IdealPFdbkVariant=Disabled  SatFdbkVariant=Disabled  DerivativeFilterVariant=Disabled  NVariant=Disabled  NCopyVariant=Disabled_SignalSpec  FilterICVariant=Disabled  IntegratorICVariant=InternalICs  ExternalResetVariant=Disabled  TRSumVariant=Passthrough  SumFdbkVariant=Disabled  SumVariant=Sum_PI  TsampFilterVariant=InternalTs  TsampNgainVariant=Passthrough  TsampIntegralVariant=Passthrough  ExternalSaturationOutDataTypeStr=Inherit: Same as second input
  PID Controller2 : slpidlib/PID Controller  Controller=PI  Form=Parallel  TimeDomain=Discrete-time  UseExternalTs=off  SampleTime=Ts  IntegratorMethod=Forward Euler  FilterMethod=Forward Euler  ControllerParametersSource=internal  P=0.009  I=0  UseKiTs=off  D=0  N=100  UseFilter=on  TunerSelectOption=Transfer Function Based (PID Tuner App)  InitialConditionSource=internal  InitialConditionForIntegrator=0  InitialConditionForFilter=0  DifferentiatorICPrevScaledInput=0  ExternalReset=none  TrackingMode=off  Kt=1  LimitOutput=on  SatLimitsSource=internal  UpperSaturationLimit=0.95  LowerSaturationLimit=0  LinearizeAsGain=on  AntiWindupMode=clamping  Kb=1  LimitIntegrator=off  UpperIntegratorSaturationLimit=inf  LowerIntegratorSaturationLimit=-inf  POutMin=[]  POutMax=[]  IOutMin=[]  IOutMax=[]  DOutMin=[]  DOutMax=[]  NOutMin=[]  NOutMax=[]  SumOutMin=[]  SumOutMax=[]  SaturationOutMin=[]  SaturationOutMax=[]  PParamMin=[]  PParamMax=[]  IParamMin=[]  IParamMax=[]  DParamMin=[]  DParamMax=[]  NParamMin=[]  NParamMax=[]  KbParamMin=[]  KbParamMax=[]  KtParamMin=[]  KtParamMax=[]  KbOutMin=[]  KbOutMax=[]  KtOutMin=[]  KtOutMax=[]  IntegratorOutMin=[]  IntegratorOutMax=[]  FilterOutMin=[]  FilterOutMax=[]  SumI1OutMin=[]  SumI1OutMax=[]  SumI2OutMin=[]  SumI2OutMax=[]  SumI3OutMin=[]  SumI3OutMax=[]  SumI4OutMin=[]  SumI4OutMax=[]  SumDOutMin=[]  SumDOutMax=[]  DifferentiatorOutMin=[]  DifferentiatorOutMax=[]  FilterDiffOutCoefMin=[]  FilterDiffOutCoefMax=[]  ReciprocalOutMin=[]  ReciprocalOutMax=[]  SumDenOutMin=[]  SumDenOutMax=[]  SumNumOutMin=[]  SumNumOutMax=[]  DivideOutMin=[]  DivideOutMax=[]  UdiffTsProdOutMin=[]  UdiffTsProdOutMax=[]  NTsProdOutMin=[]  NTsProdOutMax=[]  UintegralTsProdOutMin=[]  UintegralTsProdOutMax=[]  UngainTsProdOutMin=[]  UngainTsProdOutMax=[]  ClampingZeroOutDataTypeStr=Inherit: Inherit via back propagation  ClampingZeroOutMin=[]  ClampingZeroOutMax=[]  FilterDenConstantOutDataTypeStr=Inherit: Inherit via back propagation  FilterDenConstantOutMin=[]  FilterDenConstantOutMax=[]  PCopyOutDataTypeStr=Inherit: Inherit via back propagation  PCopyOutMin=[]  PCopyOutMax=[]  NCopyOutDataTypeStr=Inherit: Inherit via back propagation  NCopyOutMin=[]  NCopyOutMax=[]  IntegratorContinuousStateAttributes=''  IntegratorStateMustResolveToSignalObject=off  IntegratorRTWStateStorageClass=Auto  FilterContinuousStateAttributes=''  FilterStateMustResolveToSignalObject=off  FilterRTWStateStorageClass=Auto  ParallelPVariant=InternalParameters  IdealPVariant=Disabled  IVariant=InternalParameters  DVariant=Disabled  IntegratorVariant=Discrete  SatVariant=Enabled  AWVariant=DiscClampingParallel  PCopyVariant=Disabled  TRVariant=Disabled  FdbkBlocksVariant=Forward  IdealPFdbkVariant=Disabled  SatFdbkVariant=Disabled  DerivativeFilterVariant=Disabled  NVariant=Disabled  NCopyVariant=Disabled_SignalSpec  FilterICVariant=Disabled  IntegratorICVariant=InternalICs  ExternalResetVariant=Disabled  TRSumVariant=Passthrough  SumFdbkVariant=Disabled  SumVariant=Sum_PI  TsampFilterVariant=InternalTs  TsampNgainVariant=Passthrough  TsampIntegralVariant=Passthrough  ExternalSaturationOutDataTypeStr=Inherit: Same as second input
  PID Controller3 : slpidlib/PID Controller  Controller=PI  Form=Parallel  TimeDomain=Discrete-time  UseExternalTs=off  SampleTime=Ts  IntegratorMethod=Forward Euler  FilterMethod=Forward Euler  ControllerParametersSource=internal  P=0.001  I=0.02  UseKiTs=off  D=0  N=100  UseFilter=on  TunerSelectOption=Transfer Function Based (PID Tuner App)  InitialConditionSource=internal  InitialConditionForIntegrator=0  InitialConditionForFilter=0  DifferentiatorICPrevScaledInput=0  ExternalReset=none  TrackingMode=off  Kt=1  LimitOutput=on  SatLimitsSource=internal  UpperSaturationLimit=0.95  LowerSaturationLimit=0  LinearizeAsGain=on  AntiWindupMode=clamping  Kb=1  LimitIntegrator=off  UpperIntegratorSaturationLimit=inf  LowerIntegratorSaturationLimit=-inf  POutMin=[]  POutMax=[]  IOutMin=[]  IOutMax=[]  DOutMin=[]  DOutMax=[]  NOutMin=[]  NOutMax=[]  SumOutMin=[]  SumOutMax=[]  SaturationOutMin=[]  SaturationOutMax=[]  PParamMin=[]  PParamMax=[]  IParamMin=[]  IParamMax=[]  DParamMin=[]  DParamMax=[]  NParamMin=[]  NParamMax=[]  KbParamMin=[]  KbParamMax=[]  KtParamMin=[]  KtParamMax=[]  KbOutMin=[]  KbOutMax=[]  KtOutMin=[]  KtOutMax=[]  IntegratorOutMin=[]  IntegratorOutMax=[]  FilterOutMin=[]  FilterOutMax=[]  SumI1OutMin=[]  SumI1OutMax=[]  SumI2OutMin=[]  SumI2OutMax=[]  SumI3OutMin=[]  SumI3OutMax=[]  SumI4OutMin=[]  SumI4OutMax=[]  SumDOutMin=[]  SumDOutMax=[]  DifferentiatorOutMin=[]  DifferentiatorOutMax=[]  FilterDiffOutCoefMin=[]  FilterDiffOutCoefMax=[]  ReciprocalOutMin=[]  ReciprocalOutMax=[]  SumDenOutMin=[]  SumDenOutMax=[]  SumNumOutMin=[]  SumNumOutMax=[]  DivideOutMin=[]  DivideOutMax=[]  UdiffTsProdOutMin=[]  UdiffTsProdOutMax=[]  NTsProdOutMin=[]  NTsProdOutMax=[]  UintegralTsProdOutMin=[]  UintegralTsProdOutMax=[]  UngainTsProdOutMin=[]  UngainTsProdOutMax=[]  ClampingZeroOutDataTypeStr=Inherit: Inherit via back propagation  ClampingZeroOutMin=[]  ClampingZeroOutMax=[]  FilterDenConstantOutDataTypeStr=Inherit: Inherit via back propagation  FilterDenConstantOutMin=[]  FilterDenConstantOutMax=[]  PCopyOutDataTypeStr=Inherit: Inherit via back propagation  PCopyOutMin=[]  PCopyOutMax=[]  NCopyOutDataTypeStr=Inherit: Inherit via back propagation  NCopyOutMin=[]  NCopyOutMax=[]  IntegratorContinuousStateAttributes=''  IntegratorStateMustResolveToSignalObject=off  IntegratorRTWStateStorageClass=Auto  FilterContinuousStateAttributes=''  FilterStateMustResolveToSignalObject=off  FilterRTWStateStorageClass=Auto  ParallelPVariant=InternalParameters  IdealPVariant=Disabled  IVariant=InternalParameters  DVariant=Disabled  IntegratorVariant=Discrete  SatVariant=Enabled  AWVariant=DiscClampingParallel  PCopyVariant=Disabled  TRVariant=Disabled  FdbkBlocksVariant=Forward  IdealPFdbkVariant=Disabled  SatFdbkVariant=Disabled  DerivativeFilterVariant=Disabled  NVariant=Disabled  NCopyVariant=Disabled_SignalSpec  FilterICVariant=Disabled  IntegratorICVariant=InternalICs  ExternalResetVariant=Disabled  TRSumVariant=Passthrough  SumFdbkVariant=Disabled  SumVariant=Sum_PI  TsampFilterVariant=InternalTs  TsampNgainVariant=Passthrough  TsampIntegralVariant=Passthrough  ExternalSaturationOutDataTypeStr=Inherit: Same as second input
  PID Controller4 : slpidlib/PID Controller  Controller=PI  Form=Parallel  TimeDomain=Discrete-time  UseExternalTs=off  SampleTime=Ts  IntegratorMethod=Forward Euler  FilterMethod=Forward Euler  ControllerParametersSource=internal  P=0.06  I=0  UseKiTs=off  D=0  N=100  UseFilter=on  TunerSelectOption=Transfer Function Based (PID Tuner App)  InitialConditionSource=internal  InitialConditionForIntegrator=0  InitialConditionForFilter=0  DifferentiatorICPrevScaledInput=0  ExternalReset=none  TrackingMode=off  Kt=1  LimitOutput=on  SatLimitsSource=internal  UpperSaturationLimit=0.95  LowerSaturationLimit=0  LinearizeAsGain=on  AntiWindupMode=clamping  Kb=1  LimitIntegrator=off  UpperIntegratorSaturationLimit=inf  LowerIntegratorSaturationLimit=-inf  POutMin=[]  POutMax=[]  IOutMin=[]  IOutMax=[]  DOutMin=[]  DOutMax=[]  NOutMin=[]  NOutMax=[]  SumOutMin=[]  SumOutMax=[]  SaturationOutMin=[]  SaturationOutMax=[]  PParamMin=[]  PParamMax=[]  IParamMin=[]  IParamMax=[]  DParamMin=[]  DParamMax=[]  NParamMin=[]  NParamMax=[]  KbParamMin=[]  KbParamMax=[]  KtParamMin=[]  KtParamMax=[]  KbOutMin=[]  KbOutMax=[]  KtOutMin=[]  KtOutMax=[]  IntegratorOutMin=[]  IntegratorOutMax=[]  FilterOutMin=[]  FilterOutMax=[]  SumI1OutMin=[]  SumI1OutMax=[]  SumI2OutMin=[]  SumI2OutMax=[]  SumI3OutMin=[]  SumI3OutMax=[]  SumI4OutMin=[]  SumI4OutMax=[]  SumDOutMin=[]  SumDOutMax=[]  DifferentiatorOutMin=[]  DifferentiatorOutMax=[]  FilterDiffOutCoefMin=[]  FilterDiffOutCoefMax=[]  ReciprocalOutMin=[]  ReciprocalOutMax=[]  SumDenOutMin=[]  SumDenOutMax=[]  SumNumOutMin=[]  SumNumOutMax=[]  DivideOutMin=[]  DivideOutMax=[]  UdiffTsProdOutMin=[]  UdiffTsProdOutMax=[]  NTsProdOutMin=[]  NTsProdOutMax=[]  UintegralTsProdOutMin=[]  UintegralTsProdOutMax=[]  UngainTsProdOutMin=[]  UngainTsProdOutMax=[]  ClampingZeroOutDataTypeStr=Inherit: Inherit via back propagation  ClampingZeroOutMin=[]  ClampingZeroOutMax=[]  FilterDenConstantOutDataTypeStr=Inherit: Inherit via back propagation  FilterDenConstantOutMin=[]  FilterDenConstantOutMax=[]  PCopyOutDataTypeStr=Inherit: Inherit via back propagation  PCopyOutMin=[]  PCopyOutMax=[]  NCopyOutDataTypeStr=Inherit: Inherit via back propagation  NCopyOutMin=[]  NCopyOutMax=[]  IntegratorContinuousStateAttributes=''  IntegratorStateMustResolveToSignalObject=off  IntegratorRTWStateStorageClass=Auto  FilterContinuousStateAttributes=''  FilterStateMustResolveToSignalObject=off  FilterRTWStateStorageClass=Auto  ParallelPVariant=InternalParameters  IdealPVariant=Disabled  IVariant=InternalParameters  DVariant=Disabled  IntegratorVariant=Discrete  SatVariant=Enabled  AWVariant=DiscClampingParallel  PCopyVariant=Disabled  TRVariant=Disabled  FdbkBlocksVariant=Forward  IdealPFdbkVariant=Disabled  SatFdbkVariant=Disabled  DerivativeFilterVariant=Disabled  NVariant=Disabled  NCopyVariant=Disabled_SignalSpec  FilterICVariant=Disabled  IntegratorICVariant=InternalICs  ExternalResetVariant=Disabled  TRSumVariant=Passthrough  SumFdbkVariant=Disabled  SumVariant=Sum_PI  TsampFilterVariant=InternalTs  TsampNgainVariant=Passthrough  TsampIntegralVariant=Passthrough  ExternalSaturationOutDataTypeStr=Inherit: Same as second input
  Relational Operator1 : RelationalOperator  OutDataTypeStr=boolean  InputSameDT=off
  Repeating Sequence2 : simulink/Sources/Repeating Sequence  rep_seq_t=[0 Ts/2 Ts]  rep_seq_y=[0 1 0]
  Scope : Scope
  Scope1 : Scope  NumInputPorts=4
  Sum7 : Sum  Inputs=|+-
  powergui : spspowerguiLib/powergui  Priority=1  SimulationMode=Discrete  SampleTime=1e-5  frequency=60  Iterations=50  frequencyindice=0  Pbase=100e6  ErrMax=1e-4  UnitsV=kV  UnitsW=MW  buscounter=0  FunctionMessages=off  echomessages=off  EnableUseOfTLC=off  CurrentSourceSwitches=off  DisableSnubberDevices=off  DisableRonSwitches=off  DisableVfSwitches=off  DisplayEquations=off  AutomaticDiscreteSolvers=off  SolverType=Tustin/Backward Euler (TBE)  Interpol=off  ExternalGateDelay=off  methode=off  Ts=100  x0status=blocks  SPID=on  SwTol=0  HookPort=off  NonlinearTolerance=1e-4  nMaxIteration=100  ContinueOnMaxIteration=off  RestoreLinks=warning  ResistiveCurrentMeasurement=off  Frange=[0:2:500]  Ylog=off  Xlog=on  ShowGrid=off  save=off  variable=ZData  structure=0  ZoomFFT=off  StartTime=0.0  cycles=1  DisplayStyle=1  fundamental=60  FreqAxis=off  MaxFrequency=1000  frequencyindicesteady=1  RmsSteady=1  display=off
  Pulse : Outport
  wires:
  Is/1 -> Scope1/2, Sum7/2
  Pot_ref/1 -> Divide/1
  Repeating Sequence2/1 -> Relational Operator1/2
  Relational Operator1/1 -> Scope/1, Pulse/1  "S2"
  Sum7/1 -> PID Controller4/1, Scope1/3  "I_B_Actuation"
  PID Controller4/1 -> Scope1/4, Relational Operator1/1  "I_B_Actuation"
  Divide/1 -> Scope1/1, Sum7/1
  Vs/1 -> Divide/2

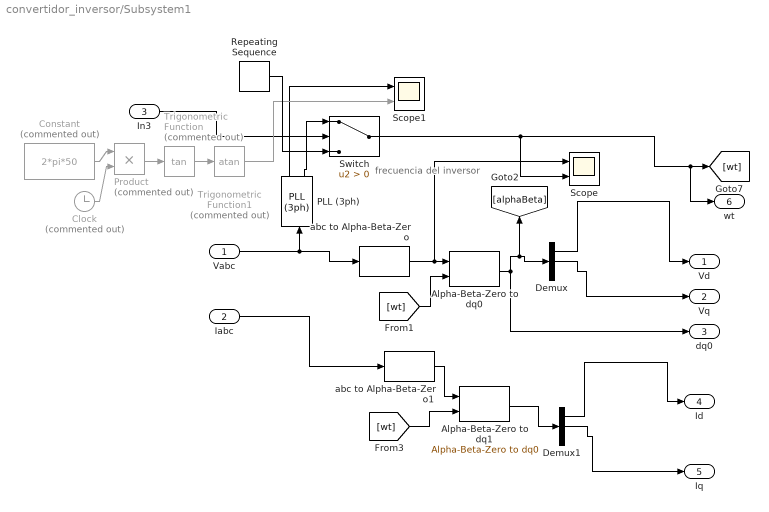
== system convertidor_inversor/Subsystem1 ==
  note: frecuencia del inversor
  Vabc : Inport
  Iabc : Inport  Port=2
  In3 : Inport  Port=3
  Alpha-Beta-Zero to dq0 : spsAlphaBetaZerotodq0Lib/Alpha-Beta-Zero to dq0  Alignment=90 degrees behind phase A axis
  Alpha-Beta-Zero to dq1 : spsAlphaBetaZerotodq0Lib/Alpha-Beta-Zero to dq0  Alignment=90 degrees behind phase A axis
  Clock : Clock  Commented=on
  Constant : Constant  Commented=on  Value=2*pi*50
  Demux : Demux  Outputs=3
  Demux1 : Demux  Outputs=3
  PLL (3ph) : spsPLL3phLib/PLL (3ph)  Fmin=45  Par_Init=[0, 50]  ParK=[180, 3200, 1]  TcD=1e-4  MaxRateChangeFreq=12  FilterCutOffFreq=25  Ts=0  AGC=on
  Product : Product  Commented=on
  Repeating Sequence : simulink/Sources/Repeating Sequence  rep_seq_t=[0 1/50]  rep_seq_y=[0 2*pi]
  Scope : Scope  NumInputPorts=2
  Scope1 : Scope  NumInputPorts=2
  Switch : Switch  Criteria=u2 > Threshold  SaturateOnIntegerOverflow=off  InputSameDT=off
  Trigonometric Function : Trigonometry  Commented=on  Operator=tan
  Trigonometric Function1 : Trigonometry  Commented=on  Operator=atan
  abc to Alpha-Beta-Zero : spsabctoAlphaBetaZeroLib/abc to Alpha-Beta-Zero
  abc to Alpha-Beta-Zero1 : spsabctoAlphaBetaZeroLib/abc to Alpha-Beta-Zero
  Vd : Outport
  Vq : Outport  Port=2
  dq0 : Outport  Port=3
  Id : Outport  Port=4
  Iq : Outport  Port=5
  wt : Outport  Port=6
  wires:
  Demux/2 -> Vq/1
  Demux1/1 -> Id/1
  Demux1/2 -> Iq/1
  Alpha-Beta-Zero to dq0/1 -> dq0/1, Demux/1, [alphaBeta]
  abc to Alpha-Beta-Zero/1 -> Scope/1, Alpha-Beta-Zero to dq0/1
  abc to Alpha-Beta-Zero1/1 -> Alpha-Beta-Zero to dq1/1
  Alpha-Beta-Zero to dq1/1 -> Demux1/1
  [wt] -> Alpha-Beta-Zero to dq0/2
  Vabc/1 -> abc to Alpha-Beta-Zero/1, PLL (3ph)/1
  [wt] -> Alpha-Beta-Zero to dq1/2
  Demux/1 -> Vd/1
  Iabc/1 -> abc to Alpha-Beta-Zero1/1
  PLL (3ph)/1 -> Scope1/1
  In3/1 -> Switch/2
  Product/1 -> Trigonometric Function/1
  Constant/1 -> Product/1
  Clock/1 -> Product/2
  Trigonometric Function/1 -> Trigonometric Function1/1
  Trigonometric Function1/1 -> Scope1/2
  Repeating Sequence/1 -> Switch/3
  PLL (3ph)/2 -> Switch/1
  Switch/1 -> Scope/2, wt/1, [wt]

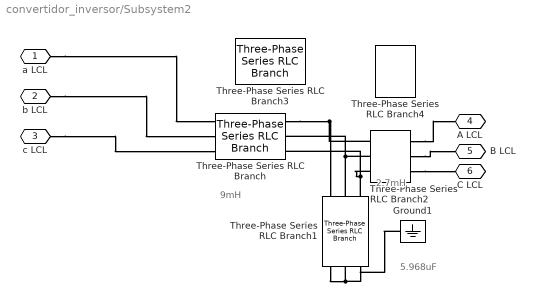
== system convertidor_inversor/Subsystem2 ==
  note: 5.968uF
  note: 9mH
  note: 2.7mH
  Ground1 : spsGroundLib/Ground  LConnTagsString=a
  Three-Phase Series RLC Branch : spsThreePhaseSeriesRLCBranchLib/Three-Phase Series RLC Branch  LConnTagsString=A|B|C  RConnTagsString=A|B|C  BranchType=L  Resistance=1  Inductance=4.186e-3  Capacitance=1e-6  Measurements=None
  Three-Phase Series RLC Branch1 : spsThreePhaseSeriesRLCBranchLib/Three-Phase Series RLC Branch  LConnTagsString=A|B|C  RConnTagsString=A|B|C  BranchType=C  Resistance=1  Inductance=1e-3  Capacitance=1.8236e-5  Measurements=None
  Three-Phase Series RLC Branch2 : spsThreePhaseSeriesRLCBranchLib/Three-Phase Series RLC Branch  LConnTagsString=A|B|C  RConnTagsString=A|B|C  BranchType=L  Resistance=1  Inductance=1.186e-3  Capacitance=1e-6  Measurements=None
  Three-Phase Series RLC Branch3 : spsThreePhaseSeriesRLCBranchLib/Three-Phase Series RLC Branch  LConnTagsString=A|B|C  RConnTagsString=A|B|C  BranchType=L  Resistance=1  Inductance=3.186e-3  Capacitance=1e-6  Measurements=None
  Three-Phase Series RLC Branch4 : spsThreePhaseSeriesRLCBranchLib/Three-Phase Series RLC Branch  LConnTagsString=A|B|C  RConnTagsString=A|B|C  BranchType=L  Resistance=1  Inductance=1.186e-3  Capacitance=1e-6  Measurements=None
  a LCL : PMIOPort  Side=Right
  "b LCL " : PMIOPort  Port=2  Side=Right
  c LCL : PMIOPort  Port=3  Side=Right
  A LCL : PMIOPort  Port=4  Side=Left
  B LCL : PMIOPort  Port=5  Side=Left
  C LCL : PMIOPort  Port=6  Side=Left
  connections:
  Three-Phase Series RLC Branch1/RConn2 -- Ground1/LConn1 -- Three-Phase Series RLC Branch1/RConn3 -- Three-Phase Series RLC Branch1/RConn1
  Three-Phase Series RLC Branch/LConn1 -- Three-Phase Series RLC Branch2/RConn1 -- Three-Phase Series RLC Branch1/LConn1
  Three-Phase Series RLC Branch1/LConn2 -- Three-Phase Series RLC Branch2/RConn2 -- Three-Phase Series RLC Branch/LConn2
  c LCL/RConn1 -- Three-Phase Series RLC Branch/RConn3
  Three-Phase Series RLC Branch1/LConn3 -- Three-Phase Series RLC Branch2/RConn3 -- Three-Phase Series RLC Branch/LConn3
  a LCL/RConn1 -- Three-Phase Series RLC Branch/RConn1
  "b LCL "/RConn1 -- Three-Phase Series RLC Branch/RConn2
  Three-Phase Series RLC Branch2/LConn2 -- B LCL/RConn1
  Three-Phase Series RLC Branch2/LConn1 -- A LCL/RConn1
  Three-Phase Series RLC Branch2/LConn3 -- C LCL/RConn1
